simulink model "BFB"  (Simulink 7.8)
settings: Solver=FixedStepDiscrete  StartTime=0.0  StopTime=1  FixedStep=0.1  RelTol=1e-5  AbsTol=1e-5
undefined symbols (not defined in the file): up
settings Model: Creator=pmahapatra  LastModifiedBy=pmahapatra
settings OptimizationCC: BlockReduction=off  BooleanDataType=off  InlineInvariantSignals=on  InitFltsAndDblsToZero=on
settings DebuggingCC: SaveWithParameterizedLinksMsg=none  SignalResolutionControl=TryResolveAllWithWarning  SolverPrmCheckMsg=none  MultiTaskDSMMsg=warning  MultiTaskCondExecSysMsg=none  FcnCallInpInsideContextMsg=Use local settings  StrictBusMsg=None
settings RTWCC: IncludeERTFirstTime=on
settings GRTTargetCC: TargetFcnLib=ansi_tfl_tmw.mat

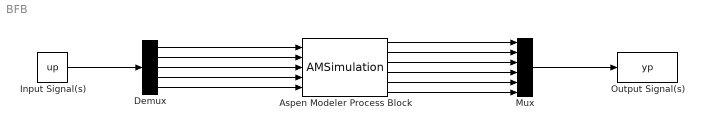
== system BFB ==
  Aspen Modeler Process Block : M-S-Function  LoadFcn=|  FunctionName=AMSimulation  Parameters="'C:\\Program Files\\CCSI\\DRMBuilder\\Examples\\BFB\\BFB.acmf','ACM Application',5,'ADSB.GasIn.F|kmol/hr\\ADSB.GasIn.T|C\\ZCO2\\ADSA.SorbIn.Fm|kg/hr\\ADSA.SorbIn.T|C',6,'CO2Removal\\STACK.Out2.F|kmol/hr\\STACK.Out2.T|C\\STACK.Out2.z(\"CO2\")|kmol/kmol\\VALVE4.Out2.Fm|kg/hr\\VALVE4.Out2.T|C',true,false,false"
      | LoadModel=actxserver('AMSimulation.Control');
      | invoke(LoadModel,'LoadModel',get_param(gcb,'Parameters'),pwd);
      | LoadModel.delete;
      settings: DeleteFcn=|
      | CloseModel=actxserver('AMSimulation.Control');
      | invoke(CloseModel,'CloseModel',get_param(gcb,'Parameters'));
      | CloseModel.delete;
      settings: OpenFcn=|
      | SetupGUI=actxserver('AMSimulation.Setup');
      | NewParam=invoke(SetupGUI,'SetupModel',get_param(gcb,'Parameters'),pwd,get_param(gcb,'Name'));
      | set_param(gcb,'Parameters',NewParam);
      | SetupGUI.delete;
  Demux : Demux  Outputs=5
  Input Signal(s) : Constant  Value=up
  Mux : Mux  Inputs=6
  Output Signal(s) : ToWorkspace  VariableName=yp  SampleTime=-1  SaveFormat=Array
  wires:
  Demux/1 -> Aspen Modeler Process Block/1
  Input Signal(s)/1 -> Demux/1
  Aspen Modeler Process Block/1 -> Mux/1
  Mux/1 -> Output Signal(s)/1
  Demux/2 -> Aspen Modeler Process Block/2
  Demux/3 -> Aspen Modeler Process Block/3
  Demux/4 -> Aspen Modeler Process Block/4
  Demux/5 -> Aspen Modeler Process Block/5
  Aspen Modeler Process Block/2 -> Mux/2
  Aspen Modeler Process Block/3 -> Mux/3
  Aspen Modeler Process Block/4 -> Mux/4
  Aspen Modeler Process Block/5 -> Mux/5
  Aspen Modeler Process Block/6 -> Mux/6
